simulink model "EPT"  (R2019b)
settings: Solver=FixedStepDiscrete  StartTime=0.0  StopTime=5  FixedStep=0.005  RelTol=1e-3  EnableMultiTasking=on
PreLoadFcn:
  | try, model_open; catch, disp('Error occurred while executing model pre-load callback: model_open.m'); disp('Please assure that the MATLAB working directory is set to the model directory before opening.'); end
InitFcn:
  | try, model_open; catch, end
undefined symbols (not defined in the file or in its folder): Bridge, GCM, H, ln, raptor_get_param_eval, raptor_get_safe_string, raptor_xcp_function
libraries: Raptor_lib x2810, simulink x374, hdlsllib x19
(part 11 of 45)

== system EPT/LED_Status/DualLED_Funny/LED_Status/10Hz ==
  Trigger : TriggerPort  VariantControl=Variant  PortDimensions=1
  NOT : Logic  Operator=NOT  IconShape=distinctive  AllPortsSameDT=off  OutDataTypeStr=boolean
  raptor_data_def : Raptor_lib/Data Storage/raptor_data_def  dataName='Flag_LED_10Hz'  initValue=0  dataType=boolean  storage=Volatile (RAM)  calVisible=on  calType=Measurement  calDispType=Number  calEnum={'False', 'True'}  calGain=1.0  calOffset=0  calMin=-inf  calMax=inf  calFormat='-1'  calUnit=''  calHelp=''  calAccess=1  calFunction=raptor_xcp_function(gcb)  calDispHeaders=off  calColHeaders={'Col1' 'Col2' 'Col3'}  calRowHeaders={'Row1' 'Row2' 'Row3'}
      settings: SourceProductName=Raptor
  raptor_data_read : Raptor_lib/Data Storage/raptor_data_read  dataName='Flag_LED_10Hz'  dataShape=Scalar  idxSource=Input  idxRow=1  idxCol=1
      settings: SourceProductName=Raptor
  raptor_data_write1 : Raptor_lib/Data Storage/raptor_data_write  dataName='Flag_LED_10Hz'  dataShape=Scalar  idxSource=Input Port  idxRow=1  idxCol=1
      settings: SourceProductName=Raptor
  wires:
  NOT/1 -> raptor_data_write1/1
  raptor_data_read/1 -> NOT/1

== system EPT/LED_Status/DualLED_Funny/LED_Status/1Hz ==
  Trigger : TriggerPort  VariantControl=Variant  PortDimensions=1
  NOT : Logic  Operator=NOT  IconShape=distinctive  AllPortsSameDT=off  OutDataTypeStr=boolean
  raptor_data_def : Raptor_lib/Data Storage/raptor_data_def  dataName='Flag_LED_1Hz'  initValue=0  dataType=boolean  storage=Volatile (RAM)  calVisible=on  calType=Measurement  calDispType=Number  calEnum={'False', 'True'}  calGain=1.0  calOffset=0  calMin=-inf  calMax=inf  calFormat='-1'  calUnit=''  calHelp=''  calAccess=1  calFunction=raptor_xcp_function(gcb)  calDispHeaders=off  calColHeaders={'Col1' 'Col2' 'Col3'}  calRowHeaders={'Row1' 'Row2' 'Row3'}
      settings: SourceProductName=Raptor
  raptor_data_read : Raptor_lib/Data Storage/raptor_data_read  dataName='Flag_LED_1Hz'  dataShape=Scalar  idxSource=Input  idxRow=1  idxCol=1
      settings: SourceProductName=Raptor
  raptor_data_write1 : Raptor_lib/Data Storage/raptor_data_write  dataName='Flag_LED_1Hz'  dataShape=Scalar  idxSource=Input Port  idxRow=1  idxCol=1
      settings: SourceProductName=Raptor
  wires:
  raptor_data_read/1 -> NOT/1
  NOT/1 -> raptor_data_write1/1

== system EPT/LED_Status/DualLED_Funny/LED_Status/2Hz ==
  Trigger : TriggerPort  VariantControl=Variant  PortDimensions=1
  NOT : Logic  Operator=NOT  IconShape=distinctive  AllPortsSameDT=off  OutDataTypeStr=boolean
  raptor_data_def : Raptor_lib/Data Storage/raptor_data_def  dataName='Flag_LED_2Hz'  initValue=0  dataType=boolean  storage=Volatile (RAM)  calVisible=on  calType=Measurement  calDispType=Number  calEnum={'False', 'True'}  calGain=1.0  calOffset=0  calMin=-inf  calMax=inf  calFormat='-1'  calUnit=''  calHelp=''  calAccess=1  calFunction=raptor_xcp_function(gcb)  calDispHeaders=off  calColHeaders={'Col1' 'Col2' 'Col3'}  calRowHeaders={'Row1' 'Row2' 'Row3'}
      settings: SourceProductName=Raptor
  raptor_data_read : Raptor_lib/Data Storage/raptor_data_read  dataName='Flag_LED_2Hz'  dataShape=Scalar  idxSource=Input  idxRow=1  idxCol=1
      settings: SourceProductName=Raptor
  raptor_data_write1 : Raptor_lib/Data Storage/raptor_data_write  dataName='Flag_LED_2Hz'  dataShape=Scalar  idxSource=Input Port  idxRow=1  idxCol=1
      settings: SourceProductName=Raptor
  wires:
  NOT/1 -> raptor_data_write1/1
  raptor_data_read/1 -> NOT/1

== system EPT/LED_Status/DualLED_Funny/LED_Status/4Hz ==
  Trigger : TriggerPort  VariantControl=Variant  PortDimensions=1
  NOT : Logic  Operator=NOT  IconShape=distinctive  AllPortsSameDT=off  OutDataTypeStr=boolean
  raptor_data_def : Raptor_lib/Data Storage/raptor_data_def  dataName='Flag_LED_4Hz'  initValue=0  dataType=boolean  storage=Volatile (RAM)  calVisible=on  calType=Measurement  calDispType=Number  calEnum={'False', 'True'}  calGain=1.0  calOffset=0  calMin=-inf  calMax=inf  calFormat='-1'  calUnit=''  calHelp=''  calAccess=1  calFunction=raptor_xcp_function(gcb)  calDispHeaders=off  calColHeaders={'Col1' 'Col2' 'Col3'}  calRowHeaders={'Row1' 'Row2' 'Row3'}
      settings: SourceProductName=Raptor
  raptor_data_read : Raptor_lib/Data Storage/raptor_data_read  dataName='Flag_LED_4Hz'  dataShape=Scalar  idxSource=Input  idxRow=1  idxCol=1
      settings: SourceProductName=Raptor
  raptor_data_write1 : Raptor_lib/Data Storage/raptor_data_write  dataName='Flag_LED_4Hz'  dataShape=Scalar  idxSource=Input Port  idxRow=1  idxCol=1
      settings: SourceProductName=Raptor
  wires:
  raptor_data_read/1 -> NOT/1
  NOT/1 -> raptor_data_write1/1

== system EPT/LED_Status/DualLED_Funny/LED_Status/Alarrn_LED ==
  Action Port : ActionPort  ActionPortLabel=case [ 7 ]:
  Constant1 : Constant  Value=6000
  Constant2 : Constant  Value=0
  Data Type Conversion : DataTypeConversion
  Switch : Switch  Threshold=1
  raptor_data_read : Raptor_lib/Data Storage/raptor_data_read  dataName='Flag_LED_10Hz'  dataShape=Scalar  idxSource=Input  idxRow=1  idxCol=1
      settings: SourceProductName=Raptor
  raptor_data_write : Raptor_lib/Data Storage/raptor_data_write  dataName='LED_Duty'  dataShape=Scalar  idxSource=Input Port  idxRow=1  idxCol=1
      settings: SourceProductName=Raptor
  wires:
  Data Type Conversion/1 -> raptor_data_write/1
  Switch/1 -> Data Type Conversion/1
  Constant2/1 -> Switch/3
  Constant1/1 -> Switch/1
  raptor_data_read/1 -> Switch/2

== system EPT/LED_Status/DualLED_Funny/LED_Status/Charging ==
  Action Port : ActionPort  ActionPortLabel=case [ 1 ]:
  Constant1 : Constant  Value=-6000
  Data Type Conversion : DataTypeConversion
  Product : Product
  raptor_data_read : Raptor_lib/Data Storage/raptor_data_read  dataName='Flag_LED_0_5Hz'  dataShape=Scalar  idxSource=Input  idxRow=1  idxCol=1
      settings: SourceProductName=Raptor
  raptor_data_write : Raptor_lib/Data Storage/raptor_data_write  dataName='LED_Duty'  dataShape=Scalar  idxSource=Input Port  idxRow=1  idxCol=1
      settings: SourceProductName=Raptor
  wires:
  raptor_data_read/1 -> Product/2
  Product/1 -> Data Type Conversion/1
  Constant1/1 -> Product/1
  Data Type Conversion/1 -> raptor_data_write/1

== system EPT/LED_Status/DualLED_Funny/LED_Status/CountTrigger1 ==
  Counter : Inport
  Constant1 : Constant  Value=0
  Constant3 : Constant
  CycleTrigger : Subsystem
  Switch : Switch  Threshold=1
  Unit Delay : UnitDelay  SampleTime=-1  HasFrameUpgradeWarning=on
  Tirgger : Outport  VectorParamsAs1DForOutWhenUnconnected=off
  wires:
  Switch/1 -> CycleTrigger/1(In1)
  Constant3/1 -> Switch/3
  Constant1/1 -> Switch/1
  Counter/1 -> CycleTrigger/2(In2)
  CycleTrigger/1(Trigger) -> Tirgger/1, Unit Delay/1
  Unit Delay/1 -> Switch/2

== system EPT/LED_Status/DualLED_Funny/LED_Status/CountTrigger2 ==
  Counter : Inport
  Constant1 : Constant  Value=0
  Constant3 : Constant
  CycleTrigger : Subsystem
  Switch : Switch  Threshold=1
  Unit Delay : UnitDelay  SampleTime=-1  HasFrameUpgradeWarning=on
  Tirgger : Outport  VectorParamsAs1DForOutWhenUnconnected=off
  wires:
  Unit Delay/1 -> Switch/2
  CycleTrigger/1(Trigger) -> Unit Delay/1, Tirgger/1
  Counter/1 -> CycleTrigger/2(In2)
  Constant1/1 -> Switch/1
  Constant3/1 -> Switch/3
  Switch/1 -> CycleTrigger/1(In1)

== system EPT/LED_Status/DualLED_Funny/LED_Status/CountTrigger3 ==
  Counter : Inport
  Constant1 : Constant  Value=0
  Constant3 : Constant
  CycleTrigger : Subsystem
  Switch : Switch  Threshold=1
  Unit Delay : UnitDelay  SampleTime=-1  HasFrameUpgradeWarning=on
  Tirgger : Outport  VectorParamsAs1DForOutWhenUnconnected=off
  wires:
  Unit Delay/1 -> Switch/2
  CycleTrigger/1(Trigger) -> Unit Delay/1, Tirgger/1
  Counter/1 -> CycleTrigger/2(In2)
  Constant1/1 -> Switch/1
  Constant3/1 -> Switch/3
  Switch/1 -> CycleTrigger/1(In1)

== system EPT/LED_Status/DualLED_Funny/LED_Status/CountTrigger4 ==
  Counter : Inport
  Constant1 : Constant  Value=0
  Constant3 : Constant
  CycleTrigger : Subsystem
  Switch : Switch  Threshold=1
  Unit Delay : UnitDelay  SampleTime=-1  HasFrameUpgradeWarning=on
  Tirgger : Outport  VectorParamsAs1DForOutWhenUnconnected=off
  wires:
  Unit Delay/1 -> Switch/2
  CycleTrigger/1(Trigger) -> Unit Delay/1, Tirgger/1
  Counter/1 -> CycleTrigger/2(In2)
  Constant1/1 -> Switch/1
  Constant3/1 -> Switch/3
  Switch/1 -> CycleTrigger/1(In1)

== system EPT/LED_Status/DualLED_Funny/LED_Status/CountTrigger5 ==
  Counter : Inport
  Constant1 : Constant  Value=0
  Constant3 : Constant
  CycleTrigger : Subsystem
  Switch : Switch  Threshold=1
  Unit Delay : UnitDelay  SampleTime=-1  HasFrameUpgradeWarning=on
  Tirgger : Outport  VectorParamsAs1DForOutWhenUnconnected=off
  wires:
  Switch/1 -> CycleTrigger/1(In1)
  Constant3/1 -> Switch/3
  Constant1/1 -> Switch/1
  Counter/1 -> CycleTrigger/2(In2)
  CycleTrigger/1(Trigger) -> Tirgger/1, Unit Delay/1
  Unit Delay/1 -> Switch/2

== system EPT/LED_Status/DualLED_Funny/LED_Status/CountTrigger6 ==
  Counter : Inport
  Constant1 : Constant  Value=0
  Constant3 : Constant
  CycleTrigger : Subsystem
  Switch : Switch  Threshold=1
  Unit Delay : UnitDelay  SampleTime=-1  HasFrameUpgradeWarning=on
  Tirgger : Outport  VectorParamsAs1DForOutWhenUnconnected=off
  wires:
  Switch/1 -> CycleTrigger/1(In1)
  Constant3/1 -> Switch/3
  Constant1/1 -> Switch/1
  Counter/1 -> CycleTrigger/2(In2)
  CycleTrigger/1(Trigger) -> Tirgger/1, Unit Delay/1
  Unit Delay/1 -> Switch/2

== system EPT/LED_Status/DualLED_Funny/LED_Status/D  ==
  Action Port : ActionPort  ActionPortLabel=case [ 6 ]:
  Abs : Abs
  Add1 : Sum
  Compare To Constant : simulink/Logic and Bit Operations/Compare To Constant  relop=>=  const=6000  OutDataTypeStr=boolean
  Compare To Constant1 : simulink/Logic and Bit Operations/Compare To Constant  relop=<=  const=-6000  OutDataTypeStr=boolean
  Data Type Conversion : DataTypeConversion
  Data Type Conversion1 : DataTypeConversion
  Gain2 : Gain  Gain=-1
  If1 : If  IfExpression=u1 >= 1  ShowElse=off
  Logical Operator : Logic  Operator=OR  AllPortsSameDT=off  OutDataTypeStr=boolean
  Scope1 : Scope
  Switch : Switch  Threshold=1
  Transition state : Subsystem  TreatAsAtomicUnit=on
  Unit Delay : UnitDelay  SampleTime=-1  HasFrameUpgradeWarning=on
  raptor_adjustment : Raptor_lib/Data Storage/raptor_adjustment  paramName='Cal_D_Duty_Scale'  nameSource=Parameter  initValue=30  dataType=double  storage=Calibration  calDispType=Number  calEnum={'False', 'True'}  calGain=1.0  calOffset=0.0  calMax=inf  calMin=-inf  calFormat='-1'  calUnit=''  calHelp=''  calAccess=1  calFunction=raptor_xcp_function(gcb)  calDispHeaders=off  calColHeaders={'Col1' 'Col2' 'Col3'}  calRowHeaders={'Row1' 'Row2' 'Row3'}
      settings: SourceProductName=Raptor
  raptor_data_read : Raptor_lib/Data Storage/raptor_data_read  dataName='LED_Gradient'  dataShape=Scalar  idxSource=Input  idxRow=1  idxCol=1
      settings: SourceProductName=Raptor
  raptor_data_write : Raptor_lib/Data Storage/raptor_data_write  dataName='LED_Duty'  dataShape=Scalar  idxSource=Input Port  idxRow=1  idxCol=1
      settings: SourceProductName=Raptor
  wires:
  Abs/1 -> Data Type Conversion/1
  If1/1 -> Transition state/Action
  Compare To Constant/1 -> Logical Operator/1
  Switch/1 -> Add1/2
  Compare To Constant1/1 -> Logical Operator/2
  Gain2/1 -> Switch/1
  Add1/1 -> Compare To Constant/1, Compare To Constant1/1, Scope1/1, Unit Delay/1, Abs/1
  raptor_adjustment/1 -> Gain2/1, Switch/3
  Data Type Conversion/1 -> raptor_data_write/1
  raptor_data_read/1 -> Switch/2
  Logical Operator/1 -> Data Type Conversion1/1
  Unit Delay/1 -> Add1/1
  Data Type Conversion1/1 -> If1/1

== system EPT/LED_Status/DualLED_Funny/LED_Status/EVSE Conected ==
  Action Port : ActionPort  ActionPortLabel=case [ 2 ]:
  Abs : Abs
  Add1 : Sum
  Compare To Constant : simulink/Logic and Bit Operations/Compare To Constant  relop=>=  const=6000  OutDataTypeStr=boolean
  Compare To Constant1 : simulink/Logic and Bit Operations/Compare To Constant  relop=<=  const=-6000  OutDataTypeStr=boolean
  Constant5 : Constant  Value=30
  Data Type Conversion : DataTypeConversion
  Data Type Conversion1 : DataTypeConversion
  Gain1 : Gain  Gain=-1
  Gain2 : Gain  Gain=-1
  If1 : If  IfExpression=u1 >= 1  ShowElse=off
  Logical Operator : Logic  Operator=OR  AllPortsSameDT=off  OutDataTypeStr=boolean
  Scope1 : Scope
  Switch : Switch  Threshold=1
  Transition state : Subsystem  TreatAsAtomicUnit=on
  Unit Delay : UnitDelay  SampleTime=-1  HasFrameUpgradeWarning=on
  raptor_data_read : Raptor_lib/Data Storage/raptor_data_read  dataName='LED_Gradient'  dataShape=Scalar  idxSource=Input  idxRow=1  idxCol=1
      settings: SourceProductName=Raptor
  raptor_data_write : Raptor_lib/Data Storage/raptor_data_write  dataName='LED_Duty'  dataShape=Scalar  idxSource=Input Port  idxRow=1  idxCol=1
      settings: SourceProductName=Raptor
  wires:
  Gain1/1 -> Data Type Conversion/1
  Data Type Conversion/1 -> raptor_data_write/1
  Abs/1 -> Gain1/1
  Compare To Constant1/1 -> Logical Operator/2
  Constant5/1 -> Gain2/1, Switch/3
  Gain2/1 -> Switch/1
  Add1/1 -> Compare To Constant/1, Compare To Constant1/1, Scope1/1, Unit Delay/1, Abs/1
  Unit Delay/1 -> Add1/1
  Logical Operator/1 -> Data Type Conversion1/1
  raptor_data_read/1 -> Switch/2
  Compare To Constant/1 -> Logical Operator/1
  If1/1 -> Transition state/Action
  Switch/1 -> Add1/2
  Data Type Conversion1/1 -> If1/1

== system EPT/LED_Status/DualLED_Funny/LED_Status/N ==
  Action Port : ActionPort  ActionPortLabel=case [ 5 ]:
  Constant1 : Constant  Value=6000
  Data Type Conversion : DataTypeConversion
  Product : Product  Inputs=3
  raptor_data_read : Raptor_lib/Data Storage/raptor_data_read  dataName='Flag_LED_0_5Hz'  dataShape=Scalar  idxSource=Input  idxRow=1  idxCol=1
      settings: SourceProductName=Raptor
  raptor_data_read1 : Raptor_lib/Data Storage/raptor_data_read  dataName='Flag_LED_2Hz'  dataShape=Scalar  idxSource=Input  idxRow=1  idxCol=1
      settings: SourceProductName=Raptor
  raptor_data_write : Raptor_lib/Data Storage/raptor_data_write  dataName='LED_Duty'  dataShape=Scalar  idxSource=Input Port  idxRow=1  idxCol=1
      settings: SourceProductName=Raptor
  wires:
  raptor_data_read/1 -> Product/2
  Product/1 -> Data Type Conversion/1
  Constant1/1 -> Product/1
  Data Type Conversion/1 -> raptor_data_write/1
  raptor_data_read1/1 -> Product/3

== system EPT/LED_Status/DualLED_Funny/LED_Status/No Mode ==
  Action Port : ActionPort  ActionPortLabel=case [ 0 ]:
  Data Type Conversion : DataTypeConversion
  Switch : Switch  Criteria=u2 > Threshold
  raptor_adjustment : Raptor_lib/Data Storage/raptor_adjustment  paramName='Cal_No_Mode_G'  nameSource=Parameter  initValue=-1000  dataType=double  storage=Calibration  calDispType=Number  calEnum={'False', 'True'}  calGain=1.0  calOffset=0.0  calMax=inf  calMin=-inf  calFormat='-1'  calUnit=''  calHelp=''  calAccess=1  calFunction=raptor_xcp_function(gcb)  calDispHeaders=off  calColHeaders={'Col1' 'Col2' 'Col3'}  calRowHeaders={'Row1' 'Row2' 'Row3'}
      settings: SourceProductName=Raptor
  raptor_adjustment1 : Raptor_lib/Data Storage/raptor_adjustment  paramName='Cal_No_Mode_R'  nameSource=Parameter  initValue=3000  dataType=double  storage=Calibration  calDispType=Number  calEnum={'False', 'True'}  calGain=1.0  calOffset=0.0  calMax=inf  calMin=-inf  calFormat='-1'  calUnit=''  calHelp=''  calAccess=1  calFunction=raptor_xcp_function(gcb)  calDispHeaders=off  calColHeaders={'Col1' 'Col2' 'Col3'}  calRowHeaders={'Row1' 'Row2' 'Row3'}
      settings: SourceProductName=Raptor
  raptor_data_read : Raptor_lib/Data Storage/raptor_data_read  dataName='Flag_LED_100Hz'  dataShape=Scalar  idxSource=Input  idxRow=1  idxCol=1
      settings: SourceProductName=Raptor
  raptor_data_write : Raptor_lib/Data Storage/raptor_data_write  dataName='LED_Duty'  dataShape=Scalar  idxSource=Input Port  idxRow=1  idxCol=1
      settings: SourceProductName=Raptor
  wires:
  Data Type Conversion/1 -> raptor_data_write/1
  Switch/1 -> Data Type Conversion/1
  raptor_adjustment/1 -> Switch/1
  raptor_adjustment1/1 -> Switch/3
  raptor_data_read/1 -> Switch/2

== system EPT/LED_Status/DualLED_Funny/LED_Status/P ==
  Action Port : ActionPort  ActionPortLabel=case [ 3 ]:
  Constant1 : Constant  Value=6000
  Data Type Conversion : DataTypeConversion
  Product : Product
  raptor_data_read : Raptor_lib/Data Storage/raptor_data_read  dataName='Flag_LED_0_5Hz'  dataShape=Scalar  idxSource=Input  idxRow=1  idxCol=1
      settings: SourceProductName=Raptor
  raptor_data_write : Raptor_lib/Data Storage/raptor_data_write  dataName='LED_Duty'  dataShape=Scalar  idxSource=Input Port  idxRow=1  idxCol=1
      settings: SourceProductName=Raptor
  wires:
  Data Type Conversion/1 -> raptor_data_write/1
  Constant1/1 -> Product/1
  Product/1 -> Data Type Conversion/1
  raptor_data_read/1 -> Product/2

== system EPT/LED_Status/DualLED_Funny/LED_Status/R ==
  Action Port : ActionPort  ActionPortLabel=case [ 4 ]:
  Abs : Abs
  Add1 : Sum
  Add2 : Sum
  Compare To Constant : simulink/Logic and Bit Operations/Compare To Constant  relop=>=  const=6000  OutDataTypeStr=boolean
  Compare To Constant1 : simulink/Logic and Bit Operations/Compare To Constant  relop=<=  const=3000  OutDataTypeStr=boolean
  Data Type Conversion : DataTypeConversion
  Data Type Conversion1 : DataTypeConversion
  Gain2 : Gain  Gain=-1
  If1 : If  IfExpression=u1 >= 1  ShowElse=off
  Logical Operator : Logic  Operator=OR  AllPortsSameDT=off  OutDataTypeStr=boolean
  Scope1 : Scope
  Switch : Switch  Threshold=1
  Transition state : Subsystem  TreatAsAtomicUnit=on
  Unit Delay : UnitDelay  SampleTime=-1  HasFrameUpgradeWarning=on
  raptor_adjustment : Raptor_lib/Data Storage/raptor_adjustment  paramName='Cal_R_Duty_Scale'  nameSource=Parameter  initValue=100  dataType=double  storage=Calibration  calDispType=Number  calEnum={'False', 'True'}  calGain=1.0  calOffset=0.0  calMax=inf  calMin=-inf  calFormat='-1'  calUnit=''  calHelp=''  calAccess=1  calFunction=raptor_xcp_function(gcb)  calDispHeaders=off  calColHeaders={'Col1' 'Col2' 'Col3'}  calRowHeaders={'Row1' 'Row2' 'Row3'}
      settings: SourceProductName=Raptor
  raptor_adjustment1 : Raptor_lib/Data Storage/raptor_adjustment  paramName='Cal_R_Base_Duty'  nameSource=Parameter  initValue=1000  dataType=double  storage=Calibration  calDispType=Number  calEnum={'False', 'True'}  calGain=1.0  calOffset=0.0  calMax=inf  calMin=-inf  calFormat='-1'  calUnit=''  calHelp=''  calAccess=1  calFunction=raptor_xcp_function(gcb)  calDispHeaders=off  calColHeaders={'Col1' 'Col2' 'Col3'}  calRowHeaders={'Row1' 'Row2' 'Row3'}
      settings: SourceProductName=Raptor
  raptor_data_read : Raptor_lib/Data Storage/raptor_data_read  dataName='LED_Gradient'  dataShape=Scalar  idxSource=Input  idxRow=1  idxCol=1
      settings: SourceProductName=Raptor
  raptor_data_write : Raptor_lib/Data Storage/raptor_data_write  dataName='LED_Duty'  dataShape=Scalar  idxSource=Input Port  idxRow=1  idxCol=1
      settings: SourceProductName=Raptor
  wires:
  Data Type Conversion1/1 -> If1/1
  Unit Delay/1 -> Add1/1
  Logical Operator/1 -> Data Type Conversion1/1
  raptor_data_read/1 -> Switch/2
  raptor_adjustment/1 -> Switch/3, Gain2/1
  Add1/1 -> Add2/1, Unit Delay/1, Scope1/1
  Gain2/1 -> Switch/1
  Compare To Constant1/1 -> Logical Operator/2
  Switch/1 -> Add1/2
  Compare To Constant/1 -> Logical Operator/1
  If1/1 -> Transition state/Action
  Abs/1 -> Data Type Conversion/1
  Data Type Conversion/1 -> raptor_data_write/1
  Add2/1 -> Compare To Constant1/1, Compare To Constant/1, Abs/1
  raptor_adjustment1/1 -> Add2/2

== system EPT/Power Up_Down/Background/Store EEPROM Value/Subsystem ==
  Enable : EnablePort
  Add : Sum
  Constant : Constant
  raptor_data_read1 : Raptor_lib/Data Storage/raptor_data_read  dataName='EEPROM_CountTest'  dataShape=Scalar  idxSource=Input  idxRow=1  idxCol=1
      settings: SourceProductName=Raptor
  raptor_data_read2 : Raptor_lib/Data Storage/raptor_data_read  dataName='EPT_BPOBU_RCAP'  dataShape=Scalar  idxSource=Input  idxRow=1  idxCol=1
      settings: SourceProductName=Raptor
  raptor_data_write1 : Raptor_lib/Data Storage/raptor_data_write  dataName='EEPROM_RCAP'  dataShape=Scalar  idxSource=Input Port  idxRow=1  idxCol=1
      settings: SourceProductName=Raptor
  raptor_data_write2 : Raptor_lib/Data Storage/raptor_data_write  dataName='EEPROM_Count'  dataShape=Scalar  idxSource=Input Port  idxRow=1  idxCol=1
      settings: SourceProductName=Raptor
  wires:
  Constant/1 -> Add/2
  Add/1 -> raptor_data_write2/1
  raptor_data_read1/1 -> Add/1
  raptor_data_read2/1 -> raptor_data_write1/1

== system EPT/Power Up_Down/Background/Store EEPROM Value/Subsystem1 ==
  Enable : EnablePort
  raptor_data_read2 : Raptor_lib/Data Storage/raptor_data_read  dataName='DOD_t'  dataShape=Scalar  idxSource=Input  idxRow=1  idxCol=1
      settings: SourceProductName=Raptor
  raptor_data_write1 : Raptor_lib/Data Storage/raptor_data_write  dataName='EEPROM_DOD_t0'  dataShape=Scalar  idxSource=Input Port  idxRow=1  idxCol=1
      settings: SourceProductName=Raptor
  wires:
  raptor_data_read2/1 -> raptor_data_write1/1

== system EPT/Power Up_Down/Background/Store EEPROM Value/Subsystem2 ==
  Enable : EnablePort
  raptor_data_read2 : Raptor_lib/Data Storage/raptor_data_read  dataName='New_SOH'  dataShape=Scalar  idxSource=Input  idxRow=1  idxCol=1
      settings: SourceProductName=Raptor
  raptor_data_write1 : Raptor_lib/Data Storage/raptor_data_write  dataName='EEPROM_SOH'  dataShape=Scalar  idxSource=Input Port  idxRow=1  idxCol=1
      settings: SourceProductName=Raptor
  wires:
  raptor_data_read2/1 -> raptor_data_write1/1

== system EPT/Power Up_Down/Background/Store EEPROM Value/Subsystem3 ==
  Enable : EnablePort
  raptor_data_read2 : Raptor_lib/Data Storage/raptor_data_read  dataName='EPT_BPOBU_FCCAP'  dataShape=Scalar  idxSource=Input  idxRow=1  idxCol=1
      settings: SourceProductName=Raptor
  raptor_data_write1 : Raptor_lib/Data Storage/raptor_data_write  dataName='EEPROM_FCCAP'  dataShape=Scalar  idxSource=Input Port  idxRow=1  idxCol=1
      settings: SourceProductName=Raptor
  wires:
  raptor_data_read2/1 -> raptor_data_write1/1

== system EPT/Test/Coulomb Counting Method Test/5ms/CountTrigger3 ==
  Counter : Inport
  Constant1 : Constant  Value=0
  Constant3 : Constant
  CycleTrigger : Subsystem
  Switch : Switch  Threshold=1
  Unit Delay1 : UnitDelay  SampleTime=-1  HasFrameUpgradeWarning=on
  Unit Delay2 : UnitDelay  SampleTime=-1  HasFrameUpgradeWarning=on
  Tirgger : Outport  VectorParamsAs1DForOutWhenUnconnected=off
  wires:
  Switch/1 -> Unit Delay1/1
  Constant3/1 -> Switch/3
  Constant1/1 -> Switch/1
  Counter/1 -> CycleTrigger/2(In2)
  CycleTrigger/1(Trigger) -> Switch/2, Unit Delay2/1
  Unit Delay1/1 -> CycleTrigger/1(In1)
  Unit Delay2/1 -> Tirgger/1

== system EPT/Test/Coulomb Counting Method Test/5ms/CountTrigger4 ==
  Counter : Inport
  Constant1 : Constant  Value=0
  Constant3 : Constant
  CycleTrigger : Subsystem
  Switch : Switch  Threshold=1
  Unit Delay1 : UnitDelay  SampleTime=-1  HasFrameUpgradeWarning=on
  Unit Delay2 : UnitDelay  SampleTime=-1  HasFrameUpgradeWarning=on
  Tirgger : Outport  VectorParamsAs1DForOutWhenUnconnected=off
  wires:
  Unit Delay2/1 -> Tirgger/1
  Unit Delay1/1 -> CycleTrigger/1(In1)
  CycleTrigger/1(Trigger) -> Unit Delay2/1, Switch/2
  Counter/1 -> CycleTrigger/2(In2)
  Constant1/1 -> Switch/1
  Constant3/1 -> Switch/3
  Switch/1 -> Unit Delay1/1

== system EPT/Test/Coulomb Counting Method Test/CountTrigger/CycleTrigger ==
  In1 : Inport
  In2 : Inport  Port=2
  Add : Sum
  Add2 : Sum  Inputs=+-
  Constant2 : Constant  Value=0
  Constant3 : Constant
  Data Type Conversion1 : DataTypeConversion
  Data Type Conversion2 : DataTypeConversion
  Relational Operator1 : RelationalOperator  OutDataTypeStr=boolean  RndMeth=Simplest
  Scope1 : Scope
  Scope2 : Scope
  Switch : Switch  Threshold=1
  Unit Delay : UnitDelay  SampleTime=-1  HasFrameUpgradeWarning=on
  Trigger : Outport  VectorParamsAs1DForOutWhenUnconnected=off
  wires:
  Add/1 -> Switch/1
  In1/1 -> Data Type Conversion2/1
  Unit Delay/1 -> Add/1
  Switch/1 -> Relational Operator1/1, Scope1/1, Unit Delay/1
  Relational Operator1/1 -> Scope2/1, Trigger/1
  Data Type Conversion1/1 -> Relational Operator1/2
  Constant2/1 -> Switch/3
  Data Type Conversion2/1 -> Add/2, Switch/2
  Add2/1 -> Data Type Conversion1/1
  In2/1 -> Add2/1
  Constant3/1 -> Add2/2

== system EPT/Test/DualLEDTest/GreenBreath/Transition state ==
  Action Port : ActionPort
  NOT : Logic  Operator=NOT  IconShape=distinctive  AllPortsSameDT=off  OutDataTypeStr=boolean
  raptor_data_read : Raptor_lib/Data Storage/raptor_data_read  dataName='LED_Gradient'  dataShape=Scalar  idxSource=Input  idxRow=1  idxCol=1
      settings: SourceProductName=Raptor
  raptor_data_write : Raptor_lib/Data Storage/raptor_data_write  dataName='LED_Gradient'  dataShape=Scalar  idxSource=Input Port  idxRow=1  idxCol=1
      settings: SourceProductName=Raptor
  wires:
  NOT/1 -> raptor_data_write/1
  raptor_data_read/1 -> NOT/1

== system EPT/Test/DualLEDTest/RedBreath/Transition state ==
  Action Port : ActionPort
  NOT : Logic  Operator=NOT  IconShape=distinctive  AllPortsSameDT=off  OutDataTypeStr=boolean
  raptor_data_read : Raptor_lib/Data Storage/raptor_data_read  dataName='LED_Gradient'  dataShape=Scalar  idxSource=Input  idxRow=1  idxCol=1
      settings: SourceProductName=Raptor
  raptor_data_write : Raptor_lib/Data Storage/raptor_data_write  dataName='LED_Gradient'  dataShape=Scalar  idxSource=Input Port  idxRow=1  idxCol=1
      settings: SourceProductName=Raptor
  wires:
  NOT/1 -> raptor_data_write/1
  raptor_data_read/1 -> NOT/1

== system EPT/Test/LED For CMU/deBounce 2/CycleTrigger1 ==
  In1 : Inport
  In2 : Inport  Port=2
  Add : Sum
  Add1 : Sum
  Add2 : Sum  Inputs=+-
  Constant1 : Constant
  Constant2 : Constant  Value=0
  Constant3 : Constant
  Data Type Conversion1 : DataTypeConversion
  Data Type Conversion2 : DataTypeConversion
  Display : Display
  Relational Operator1 : RelationalOperator  OutDataTypeStr=boolean  RndMeth=Simplest
  Saturation : Saturate  UpperLimit=inf  LowerLimit=2
  Scope : Scope
  Scope1 : Scope
  Scope2 : Scope
  Switch : Switch  Threshold=1
  Unit Delay : UnitDelay  SampleTime=-1  HasFrameUpgradeWarning=on
  Unit Delay1 : UnitDelay  SampleTime=-1  HasFrameUpgradeWarning=on
  Trigger : Outport  VectorParamsAs1DForOutWhenUnconnected=off
  wires:
  Constant3/1 -> Add2/2
  In2/1 -> Saturation/1
  Add2/1 -> Data Type Conversion1/1
  Data Type Conversion2/1 -> Switch/2, Add/2
  Constant2/1 -> Switch/3
  Data Type Conversion1/1 -> Relational Operator1/2
  Relational Operator1/1 -> Trigger/1, Scope2/1
  Constant1/1 -> Add1/2
  Unit Delay1/1 -> Add1/1
  Add1/1 -> Display/1, Unit Delay1/1, Scope/1
  Switch/1 -> Unit Delay/1, Scope1/1, Relational Operator1/1
  Unit Delay/1 -> Add/1
  In1/1 -> Data Type Conversion2/1
  Add/1 -> Switch/1
  Saturation/1 -> Add2/1

== system EPT/Test/LifeCycleTest/LifeCycleDetect/Latch1 ==
  Latch : Inport
  Reset : Inport  Port=2
  Switch1 : Switch  Criteria=u2 > Threshold
  Switch3 : Switch  Criteria=u2 > Threshold
  Unit Delay1 : UnitDelay  SampleTime=-1  HasFrameUpgradeWarning=on
  Output : Outport  VectorParamsAs1DForOutWhenUnconnected=off
  wires:
  Unit Delay1/1 -> Switch1/3
  Switch3/1 -> Output/1, Unit Delay1/1
  Reset/1 -> Switch3/2
  Latch/1 -> Switch1/1, Switch1/2
  Switch1/1 -> Switch3/3

== system EPT/Test/RPB1600_Read/CountTrigger/CycleTrigger ==
  In1 : Inport
  In2 : Inport  Port=2
  Add : Sum
  Add1 : Sum
  Add2 : Sum  Inputs=+-
  Constant1 : Constant
  Constant2 : Constant  Value=0
  Constant3 : Constant
  Data Type Conversion1 : DataTypeConversion
  Data Type Conversion2 : DataTypeConversion
  Display : Display
  Relational Operator1 : RelationalOperator  OutDataTypeStr=boolean  RndMeth=Simplest
  Scope : Scope
  Scope1 : Scope
  Scope2 : Scope
  Switch : Switch  Threshold=1
  Unit Delay : UnitDelay  SampleTime=-1  HasFrameUpgradeWarning=on
  Unit Delay1 : UnitDelay  SampleTime=-1  HasFrameUpgradeWarning=on
  Trigger : Outport  VectorParamsAs1DForOutWhenUnconnected=off
  wires:
  Constant3/1 -> Add2/2
  In2/1 -> Add2/1
  Add2/1 -> Data Type Conversion1/1
  Data Type Conversion2/1 -> Switch/2, Add/2
  Constant2/1 -> Switch/3
  Data Type Conversion1/1 -> Relational Operator1/2
  Relational Operator1/1 -> Trigger/1, Scope2/1
  Constant1/1 -> Add1/2
  Unit Delay1/1 -> Add1/1
  Add1/1 -> Display/1, Unit Delay1/1, Scope/1
  Switch/1 -> Unit Delay/1, Scope1/1, Relational Operator1/1
  Unit Delay/1 -> Add/1
  In1/1 -> Data Type Conversion2/1
  Add/1 -> Switch/1

== system EPT/Test/RPB1600_Read/RPB1600_RX_20ms/Convert_Byte2Data ==
  LowByte : Inport
  HighByte : Inport  Port=2
  Offset : Inport  Port=3
  Factor : Inport  Port=4
  Add2 : Sum
  Add5 : Sum
  Constant10 : Constant  Value=256
  Data Type Conversion10 : DataTypeConversion
  Divide6 : Product  Inputs=**
  Divide9 : Product  Inputs=**
  Data(int16) : Outport  VectorParamsAs1DForOutWhenUnconnected=off
  wires:
  Divide6/1 -> Add2/2
  LowByte/1 -> Add2/1
  Divide9/1 -> Data Type Conversion10/1
  HighByte/1 -> Divide6/1
  Constant10/1 -> Divide6/2
  Add5/1 -> Divide9/1
  Add2/1 -> Add5/1
  Data Type Conversion10/1 -> Data(int16)/1
  Offset/1 -> Add5/2
  Factor/1 -> Divide9/2

== system EPT/Test/RPB1600_Read/RPB1600_RX_20ms/Subsystem ==
  Rx Data : Inport
  Task Input : Inport  Port=2
  "Task Set " : Inport  Port=3
  Delay : Delay  DelayLength=1
  Relational Operator : RelationalOperator  Operator===  OutDataTypeStr=boolean  RndMeth=Simplest
  Switch : Switch  Criteria=u2 > Threshold
  Output : Outport  VectorParamsAs1DForOutWhenUnconnected=off
  wires:
  Relational Operator/1 -> Switch/2
  Switch/1 -> Output/1, Delay/1
  Delay/1 -> Switch/3
  "Task Set "/1 -> Relational Operator/2
  Task Input/1 -> Relational Operator/1
  Rx Data/1 -> Switch/1

== system EPT/Test/RPB1600_Read/RPB1600_RX_20ms/Subsystem1 ==
  Rx Data : Inport
  Task Input : Inport  Port=2
  "Task Set " : Inport  Port=3
  Delay : Delay  DelayLength=1
  Relational Operator : RelationalOperator  Operator===  OutDataTypeStr=boolean  RndMeth=Simplest
  Switch : Switch  Criteria=u2 > Threshold
  Output : Outport  VectorParamsAs1DForOutWhenUnconnected=off
  wires:
  Rx Data/1 -> Switch/1
  Task Input/1 -> Relational Operator/1
  "Task Set "/1 -> Relational Operator/2
  Delay/1 -> Switch/3
  Switch/1 -> Delay/1, Output/1
  Relational Operator/1 -> Switch/2

== system EPT/Test/RPB1600_Read/RPB1600_RX_20ms/Subsystem2 ==
  Rx Data : Inport
  Task Input : Inport  Port=2
  "Task Set " : Inport  Port=3
  Delay : Delay  DelayLength=1
  Relational Operator : RelationalOperator  Operator===  OutDataTypeStr=boolean  RndMeth=Simplest
  Switch : Switch  Criteria=u2 > Threshold
  Output : Outport  VectorParamsAs1DForOutWhenUnconnected=off
  wires:
  Relational Operator/1 -> Switch/2
  Switch/1 -> Output/1, Delay/1
  Delay/1 -> Switch/3
  "Task Set "/1 -> Relational Operator/2
  Task Input/1 -> Relational Operator/1
  Rx Data/1 -> Switch/1

== system EPT/Test/RPB1600_Read/RPB1600_RX_20ms/Subsystem3 ==
  Rx Data : Inport
  Task Input : Inport  Port=2
  "Task Set " : Inport  Port=3
  Delay : Delay  DelayLength=1
  Relational Operator : RelationalOperator  Operator===  OutDataTypeStr=boolean  RndMeth=Simplest
  Switch : Switch  Criteria=u2 > Threshold
  Output : Outport  VectorParamsAs1DForOutWhenUnconnected=off
  wires:
  Rx Data/1 -> Switch/1
  Task Input/1 -> Relational Operator/1
  "Task Set "/1 -> Relational Operator/2
  Delay/1 -> Switch/3
  Switch/1 -> Delay/1, Output/1
  Relational Operator/1 -> Switch/2

== system EPT/Test/RPB1600_Read/RPB1600_RX_20ms/Subsystem4 ==
  Rx Data : Inport
  Task Input : Inport  Port=2
  "Task Set " : Inport  Port=3
  Delay : Delay  DelayLength=1
  Relational Operator : RelationalOperator  Operator===  OutDataTypeStr=boolean  RndMeth=Simplest
  Switch : Switch  Criteria=u2 > Threshold
  Output : Outport  VectorParamsAs1DForOutWhenUnconnected=off
  wires:
  Relational Operator/1 -> Switch/2
  Switch/1 -> Output/1, Delay/1
  Delay/1 -> Switch/3
  "Task Set "/1 -> Relational Operator/2
  Task Input/1 -> Relational Operator/1
  Rx Data/1 -> Switch/1

== system EPT/Test/RPB1600_Read/RPB1600_RX_20ms/Subsystem5 ==
  Rx Data : Inport
  Task Input : Inport  Port=2
  "Task Set " : Inport  Port=3
  Delay : Delay  DelayLength=1
  Relational Operator : RelationalOperator  Operator===  OutDataTypeStr=boolean  RndMeth=Simplest
  Switch : Switch  Criteria=u2 > Threshold
  Output : Outport  VectorParamsAs1DForOutWhenUnconnected=off
  wires:
  Rx Data/1 -> Switch/1
  Task Input/1 -> Relational Operator/1
  "Task Set "/1 -> Relational Operator/2
  Delay/1 -> Switch/3
  Switch/1 -> Delay/1, Output/1
  Relational Operator/1 -> Switch/2

== system EPT/Test/RPB1600_Read/RPB1600_RX_20ms/Subsystem6 ==
  Rx Data : Inport
  Task Input : Inport  Port=2
  "Task Set " : Inport  Port=3
  Delay : Delay  DelayLength=1
  Relational Operator : RelationalOperator  Operator===  OutDataTypeStr=boolean  RndMeth=Simplest
  Switch : Switch  Criteria=u2 > Threshold
  Output : Outport  VectorParamsAs1DForOutWhenUnconnected=off
  wires:
  Relational Operator/1 -> Switch/2
  Switch/1 -> Output/1, Delay/1
  Delay/1 -> Switch/3
  "Task Set "/1 -> Relational Operator/2
  Task Input/1 -> Relational Operator/1
  Rx Data/1 -> Switch/1

== system EPT/Test/RPB1600_Read/RPB1600_RX_20ms/Subsystem7 ==
  Rx Data : Inport
  Task Input : Inport  Port=2
  "Task Set " : Inport  Port=3
  Delay : Delay  DelayLength=1
  Relational Operator : RelationalOperator  Operator===  OutDataTypeStr=boolean  RndMeth=Simplest
  Switch : Switch  Criteria=u2 > Threshold
  Output : Outport  VectorParamsAs1DForOutWhenUnconnected=off
  wires:
  Rx Data/1 -> Switch/1
  Task Input/1 -> Relational Operator/1
  "Task Set "/1 -> Relational Operator/2
  Delay/1 -> Switch/3
  Switch/1 -> Delay/1, Output/1
  Relational Operator/1 -> Switch/2

== system EPT/Test/RPB1600_Read/RPB1600_RX_20ms/Subsystem8 ==
  Rx Data : Inport
  Task Input : Inport  Port=2
  "Task Set " : Inport  Port=3
  Delay : Delay  DelayLength=1
  Relational Operator : RelationalOperator  Operator===  OutDataTypeStr=boolean  RndMeth=Simplest
  Switch : Switch  Criteria=u2 > Threshold
  Output : Outport  VectorParamsAs1DForOutWhenUnconnected=off
  wires:
  Relational Operator/1 -> Switch/2
  Switch/1 -> Output/1, Delay/1
  Delay/1 -> Switch/3
  "Task Set "/1 -> Relational Operator/2
  Task Input/1 -> Relational Operator/1
  Rx Data/1 -> Switch/1

== system EPT/Test/RPB1600_Read/RPB1600_RX_20ms/Subsystem9 ==
  Rx Data : Inport
  Task Input : Inport  Port=2
  "Task Set " : Inport  Port=3
  Delay : Delay  DelayLength=1
  Relational Operator : RelationalOperator  Operator===  OutDataTypeStr=boolean  RndMeth=Simplest
  Switch : Switch  Criteria=u2 > Threshold
  Output : Outport  VectorParamsAs1DForOutWhenUnconnected=off
  wires:
  Rx Data/1 -> Switch/1
  Task Input/1 -> Relational Operator/1
  "Task Set "/1 -> Relational Operator/2
  Delay/1 -> Switch/3
  Switch/1 -> Delay/1, Output/1
  Relational Operator/1 -> Switch/2

== system EPT/Test/RPB1600_Read/RPB1600_RX_20ms/Task Rolling ==
  Constant : Constant  Value=9
  RollingCount : Subsystem
  raptor_data_write : Raptor_lib/Data Storage/raptor_data_write  dataName='RPB1600_Task'  dataShape=Scalar  idxSource=Input Port  idxRow=1  idxCol=1
      settings: SourceProductName=Raptor
  wires:
  Constant/1 -> RollingCount/1(In1)
  RollingCount/1(Out1) -> raptor_data_write/1

== system EPT/Foreground_TimeBase_5ms/CAN/CAN1_exec/BCU vs RMDA-BMS/BCU-OBU Output-CTL  ==
  Trigger : TriggerPort  VariantControl=Variant  PortDimensions=1
  raptor_can_txmsg : Raptor_lib/CAN/raptor_can_txmsg  canDefinition=struct('dbcFile', 'BCU_OBU_HMI.dbc','message', 'BCU_OBU_OutputCTL','comment', '','signals', {{'BP_OBU_Vchg_EXP','BP_OBU_Ichg_EXP','BP_OBU_Iregen_LC','BP_OBU_Idchg_LC','BP_OBU_min_Limit','BP_OBU_Vmax_Limit'}},'enabled', [ 1 1 1 1 1 1;],'canBus', '''CAN1''','messageID', [ 1529;],'idMask', [ 536870911;],'payloadMask', [],'payloadValue', [],'period', [ 0;],'mailbox', '','queueSize', [ 1;],'label', [ 0;],'ver', [ 2;],'showID', [ 0;],'showRaw', [ 0;],'fill', [ 0;],'editID', [ 0;],'signalOrder', [ 2;])  canBus='CAN1'  queueSize=1  payloadMask=[]  payloadValue=[]  period=0  showID=0  label=0  idMask=hex2dec('1FFFFFFF')  fill=0  id=1529  showRaw=0  signalOrder=2  signalInfo={{struct('Name', 'BP_OBU_Vmax_Limit','Startbit', [ 0;],'SignalSize', [ 16;],'ByteOrder', 'BigEndian','ValueType', 'UNSIGNED','Class', 'uint16','Signed', [ 0;],'Factor', [ 0.01;],'Offset', [ 0;],'Min', [ 0;],'Max', [ 0;],'Units', '','Comment', '','StartBit', [ 8;]),struct('Name', 'BP_OBU_min_Limit','Startbit', [ 0;],'SignalSize', [ 16;],'ByteOrder', 'BigEndian','ValueType', 'UNSIGNED','Class', 'uint16','Signed', [ 0;],'Factor', [ 0.01;],'Offset', [ 0;],'Min', [ 0;],'Max', [ 0;],'Units', '','Comment', '','StartBit', [ 24;]),struct('Name', 'BP_OBU_Idchg_LC','Startbit', [ 0;],'SignalSize', [ 8;],'ByteOrder', 'BigEndian','ValueType', 'UNSIGNED','Class', 'uint8','Signed', [ 0;],'Factor', [ 2;],'Offset', [ -500;],'Min', [ 0;],'Max', [ 0;],'Units', '','Comment', '','StartBit', [ 32;]),struct('Name', 'BP_OBU_Iregen_LC','Startbit', [ 0;],'SignalSize', [ 8;],'ByteOrder', 'BigEndian','ValueType', 'UNSIGNED','Class', 'uint8','Signed', [ 0;],'Factor', [ 2;],'Offset', [ 0;],'Min', [ 0;],'Max', [ 0;],'Units', '','Comment', '','StartBit', [ 40;]),struct('Name', 'BP_OBU_Ichg_EXP','Startbit', [ 0;],'SignalSize', [ 8;],'ByteOrder', 'BigEndian','ValueType', 'UNSIGNED','Class', 'uint8','Signed', [ 0;],'Factor', [ 0.5;],'Offset', [ 0;],'Min', [ 0;],'Max', [ 0;],'Units', '','Comment', '','StartBit', [ 48;]),struct('Name', 'BP_OBU_Vchg_EXP','Startbit', [ 0;],'SignalSize', [ 8;],'ByteOrder', 'BigEndian','ValueType', 'UNSIGNED','Class', 'uint8','Signed', [ 0;],'Factor', [ 0.5;],'Offset', [ 0;],'Min', [ 0;],'Max', [ 0;],'Units', '','Comment', '','StartBit', [ 56;])}}
      settings: SourceProductName=Raptor
  raptor_data_def1 : Raptor_lib/Data Storage/raptor_data_def  dataName='BP_OBU_Vmin_Limit'  initValue=0  dataType=double  storage=Volatile (RAM)  calVisible=on  calType=Measurement  calDispType=Number  calEnum={'False', 'True'}  calGain=1.0  calOffset=0  calMin=-inf  calMax=inf  calFormat='-1'  calUnit=''  calHelp=''  calAccess=1  calFunction=raptor_xcp_function(gcb)  calDispHeaders=off  calColHeaders={'Col1' 'Col2' 'Col3'}  calRowHeaders={'Row1' 'Row2' 'Row3'}
      settings: SourceProductName=Raptor
  raptor_data_def2 : Raptor_lib/Data Storage/raptor_data_def  dataName='BP_OBU_Vmax_Limit'  initValue=0  dataType=double  storage=Volatile (RAM)  calVisible=on  calType=Measurement  calDispType=Number  calEnum={'False', 'True'}  calGain=1.0  calOffset=0  calMin=-inf  calMax=inf  calFormat='-1'  calUnit=''  calHelp=''  calAccess=1  calFunction=raptor_xcp_function(gcb)  calDispHeaders=off  calColHeaders={'Col1' 'Col2' 'Col3'}  calRowHeaders={'Row1' 'Row2' 'Row3'}
      settings: SourceProductName=Raptor
  raptor_data_def4 : Raptor_lib/Data Storage/raptor_data_def  dataName='BP_OBU_Vchg_EXP'  initValue=0  dataType=double  storage=Volatile (RAM)  calVisible=on  calType=Measurement  calDispType=Number  calEnum={'False', 'True'}  calGain=1.0  calOffset=0  calMin=-inf  calMax=inf  calFormat='-1'  calUnit=''  calHelp=''  calAccess=1  calFunction=raptor_xcp_function(gcb)  calDispHeaders=off  calColHeaders={'Col1' 'Col2' 'Col3'}  calRowHeaders={'Row1' 'Row2' 'Row3'}
      settings: SourceProductName=Raptor
  raptor_data_read1 : Raptor_lib/Data Storage/raptor_data_read  dataName='Ichg_cc_exp'  dataShape=Scalar  idxSource=Input  idxRow=1  idxCol=1
      settings: SourceProductName=Raptor
  raptor_data_read2 : Raptor_lib/Data Storage/raptor_data_read  dataName='Iregen_con_exp'  dataShape=Scalar  idxSource=Input  idxRow=1  idxCol=1
      settings: SourceProductName=Raptor
  raptor_data_read3 : Raptor_lib/Data Storage/raptor_data_read  dataName='BP_OBU_Vchg_EXP'  dataShape=Scalar  idxSource=Input  idxRow=1  idxCol=1
      settings: SourceProductName=Raptor
  raptor_data_read4 : Raptor_lib/Data Storage/raptor_data_read  dataName='Idchg_con_exp'  dataShape=Scalar  idxSource=Input  idxRow=1  idxCol=1
      settings: SourceProductName=Raptor
  raptor_data_read5 : Raptor_lib/Data Storage/raptor_data_read  dataName='BP_OBU_Vmin_Limit'  dataShape=Scalar  idxSource=Input  idxRow=1  idxCol=1
      settings: SourceProductName=Raptor
  raptor_data_read6 : Raptor_lib/Data Storage/raptor_data_read  dataName='BP_OBU_Vmax_Limit'  dataShape=Scalar  idxSource=Input  idxRow=1  idxCol=1
      settings: SourceProductName=Raptor
  wires:
  raptor_data_read3/1 -> raptor_can_txmsg/1
  raptor_data_read1/1 -> raptor_can_txmsg/2
  raptor_data_read4/1 -> raptor_can_txmsg/4
  raptor_data_read5/1 -> raptor_can_txmsg/5
  raptor_data_read6/1 -> raptor_can_txmsg/6
  raptor_data_read2/1 -> raptor_can_txmsg/3

== system EPT/Foreground_TimeBase_5ms/CAN/CAN1_exec/BCU vs RMDA-BMS/BCU-OBU Output-EW Code ==
  Trigger : TriggerPort  VariantControl=Variant  PortDimensions=1
  raptor_can_txmsg : Raptor_lib/CAN/raptor_can_txmsg  canDefinition=struct('dbcFile', 'BCU_OBU_HMI.dbc','message', 'BCU_OBU_Output_EW_Code','comment', '','signals', {{'BP_OBU_Fault_G5','BP_OBU_Fault_G4','BP_OBU_Fault_G3','BP_OBU_Fault_G2','BP_OBU_Fault_G1','BP_OBU_Warning_G3','BP_OBU_Warning_G2','BP_OBU_Warning_G1'}},'enabled', [ 1 1 1 1 1 1 1 1;],'canBus', '''CAN1''','messageID', [ 1524;],'idMask', [ 536870911;],'payloadMask', [],'payloadValue', [],'period', [ 0;],'mailbox', '','queueSize', [ 1;],'label', [ 0;],'ver', [ 2;],'showID', [ 0;],'showRaw', [ 0;],'fill', [ 0;],'editID', [ 0;],'signalOrder', [ 2;])  canBus='CAN1'  queueSize=1  payloadMask=[]  payloadValue=[]  period=0  showID=0  label=0  idMask=hex2dec('1FFFFFFF')  fill=0  id=1524  showRaw=0  signalOrder=2  signalInfo={{struct('Name', 'BP_OBU_Warning_G3','Startbit', [ 0;],'SignalSize', [ 8;],'ByteOrder', 'BigEndian','ValueType', 'UNSIGNED','Class', 'uint8','Signed', [ 0;],'Factor', [ 1;],'Offset', [ 0;],'Min', [ 0;],'Max', [ 0;],'Units', '','Comment', '','StartBit', [ 16;]),struct('Name', 'BP_OBU_Warning_G2','Startbit', [ 0;],'SignalSize', [ 8;],'ByteOrder', 'BigEndian','ValueType', 'UNSIGNED','Class', 'uint8','Signed', [ 0;],'Factor', [ 1;],'Offset', [ 0;],'Min', [ 0;],'Max', [ 0;],'Units', '','Comment', '','StartBit', [ 8;]),struct('Name', 'BP_OBU_Warning_G1','Startbit', [ 0;],'SignalSize', [ 8;],'ByteOrder', 'BigEndian','ValueType', 'UNSIGNED','Class', 'uint8','Signed', [ 0;],'Factor', [ 1;],'Offset', [ 0;],'Min', [ 0;],'Max', [ 0;],'Units', '','Comment', '','StartBit', [ 0;]),struct('Name', 'BP_OBU_Fault_G5','Startbit', [ 0;],'SignalSize', [ 8;],'ByteOrder', 'BigEndian','ValueType', 'UNSIGNED','Class', 'uint8','Signed', [ 0;],'Factor', [ 1;],'Offset', [ 0;],'Min', [ 0;],'Max', [ 0;],'Units', '','Comment', '','StartBit', [ 56;]),struct('Name', 'BP_OBU_Fault_G4','Startbit', [ 0;],'SignalSize', [ 8;],'ByteOrder', 'BigEndian','ValueType', 'UNSIGNED','Class', 'uint8','Signed', [ 0;],'Factor', [ 1;],'Offset', [ 0;],'Min', [ 0;],'Max', [ 0;],'Units', '','Comment', '','StartBit', [ 48;]),struct('Name', 'BP_OBU_Fault_G3','Startbit', [ 0;],'SignalSize', [ 8;],'ByteOrder', 'BigEndian','ValueType', 'UNSIGNED','Class', 'uint8','Signed', [ 0;],'Factor', [ 1;],'Offset', [ 0;],'Min', [ 0;],'Max', [ 0;],'Units', '','Comment', '','StartBit', [ 40;]),struct('Name', 'BP_OBU_Fault_G2','Startbit', [ 0;],'SignalSize', [ 8;],'ByteOrder', 'BigEndian','ValueType', 'UNSIGNED','Class', 'uint8','Signed', [ 0;],'Factor', [ 1;],'Offset', [ 0;],'Min', [ 0;],'Max', [ 0;],'Units', '','Comment', '','StartBit', [ 32;]),struct('Name', 'BP_OBU_Fault_G1','Startbit', [ 0;],'SignalSize', [ 8;],'ByteOrder', 'BigEndian','ValueType', 'UNSIGNED','Class', 'uint8','Signed', [ 0;],'Factor', [ 1;],'Offset', [ 0;],'Min', [ 0;],'Max', [ 0;],'Units', '','Comment', '','StartBit', [ 24;])}}
      settings: SourceProductName=Raptor
  raptor_data_read : Raptor_lib/Data Storage/raptor_data_read  dataName='BP_OBU_Fault_G5'  dataShape=Scalar  idxSource=Input  idxRow=1  idxCol=1
      settings: SourceProductName=Raptor
  raptor_data_read1 : Raptor_lib/Data Storage/raptor_data_read  dataName='BP_OBU_Warning_G3'  dataShape=Scalar  idxSource=Input  idxRow=1  idxCol=1
      settings: SourceProductName=Raptor
  raptor_data_read2 : Raptor_lib/Data Storage/raptor_data_read  dataName='BP_OBU_Fault_G4'  dataShape=Scalar  idxSource=Input  idxRow=1  idxCol=1
      settings: SourceProductName=Raptor
  raptor_data_read3 : Raptor_lib/Data Storage/raptor_data_read  dataName='BP_OBU_Fault_G3'  dataShape=Scalar  idxSource=Input  idxRow=1  idxCol=1
      settings: SourceProductName=Raptor
  raptor_data_read4 : Raptor_lib/Data Storage/raptor_data_read  dataName='BP_OBU_Fault_G2'  dataShape=Scalar  idxSource=Input  idxRow=1  idxCol=1
      settings: SourceProductName=Raptor
  raptor_data_read5 : Raptor_lib/Data Storage/raptor_data_read  dataName='BP_OBU_Fault_G1'  dataShape=Scalar  idxSource=Input  idxRow=1  idxCol=1
      settings: SourceProductName=Raptor
  raptor_data_read6 : Raptor_lib/Data Storage/raptor_data_read  dataName='BP_OBU_Warning_G2'  dataShape=Scalar  idxSource=Input  idxRow=1  idxCol=1
      settings: SourceProductName=Raptor
  raptor_data_read7 : Raptor_lib/Data Storage/raptor_data_read  dataName='BP_OBU_Warning_G1'  dataShape=Scalar  idxSource=Input  idxRow=1  idxCol=1
      settings: SourceProductName=Raptor
  wires:
  raptor_data_read/1 -> raptor_can_txmsg/1
  raptor_data_read2/1 -> raptor_can_txmsg/2
  raptor_data_read3/1 -> raptor_can_txmsg/3
  raptor_data_read4/1 -> raptor_can_txmsg/4
  raptor_data_read5/1 -> raptor_can_txmsg/5
  raptor_data_read1/1 -> raptor_can_txmsg/6
  raptor_data_read6/1 -> raptor_can_txmsg/7
  raptor_data_read7/1 -> raptor_can_txmsg/8

== system EPT/Foreground_TimeBase_5ms/CAN/CAN1_exec/BCU vs RMDA-BMS/BCU-OBU Status-OP G1 ==
  Trigger : TriggerPort  VariantControl=Variant  PortDimensions=1
  raptor_can_txmsg : Raptor_lib/CAN/raptor_can_txmsg  canDefinition=struct('dbcFile', 'BCU_OBU_HMI.dbc','message', 'BCU_OBU_Status_OP_G1','comment', '','signals', {{'BP_OBU_Vbus','BP_OBU_Vbatt','BP_OBU_Current'}},'enabled', [ 1 1 1;],'canBus', '''CAN1''','messageID', [ 1525;],'idMask', [ 536870911;],'payloadMask', [],'payloadValue', [],'period', [ 0;],'mailbox', '','queueSize', [ 1;],'label', [ 0;],'ver', [ 2;],'showID', [ 0;],'showRaw', [ 0;],'fill', [ 0;],'editID', [ 0;],'signalOrder', [ 2;])  canBus='CAN1'  queueSize=1  payloadMask=[]  payloadValue=[]  period=0  showID=0  label=0  idMask=hex2dec('1FFFFFFF')  fill=0  id=1525  showRaw=0  signalOrder=2  signalInfo={{struct('Name', 'BP_OBU_Current','Startbit', [ 0;],'SignalSize', [ 16;],'ByteOrder', 'BigEndian','ValueType', 'UNSIGNED','Class', 'uint16','Signed', [ 0;],'Factor', [ 0.02;],'Offset', [ -500;],'Min', [ 0;],'Max', [ 0;],'Units', '','Comment', '','StartBit', [ 8;]),struct('Name', 'BP_OBU_Vbatt','Startbit', [ 0;],'SignalSize', [ 16;],'ByteOrder', 'BigEndian','ValueType', 'UNSIGNED','Class', 'uint16','Signed', [ 0;],'Factor', [ 0.01;],'Offset', [ 0;],'Min', [ 0;],'Max', [ 0;],'Units', '','Comment', '','StartBit', [ 24;]),struct('Name', 'BP_OBU_Vbus','Startbit', [ 0;],'SignalSize', [ 16;],'ByteOrder', 'BigEndian','ValueType', 'UNSIGNED','Class', 'uint16','Signed', [ 0;],'Factor', [ 0.01;],'Offset', [ 0;],'Min', [ 0;],'Max', [ 0;],'Units', '','Comment', '','StartBit', [ 40;])}}
      settings: SourceProductName=Raptor
  raptor_data_read1 : Raptor_lib/Data Storage/raptor_data_read  dataName='EPT_BPOBU_VOLT'  dataShape=Scalar  idxSource=Input  idxRow=1  idxCol=1
      settings: SourceProductName=Raptor
  raptor_data_read2 : Raptor_lib/Data Storage/raptor_data_read  dataName='EPT_HV_BUS_VOLT'  dataShape=Scalar  idxSource=Input  idxRow=1  idxCol=1
      settings: SourceProductName=Raptor
  raptor_data_read5 : Raptor_lib/Data Storage/raptor_data_read  dataName='EPT_BPOBU_CURR'  dataShape=Scalar  idxSource=Input  idxRow=1  idxCol=1
      settings: SourceProductName=Raptor
  wires:
  raptor_data_read2/1 -> raptor_can_txmsg/1
  raptor_data_read1/1 -> raptor_can_txmsg/2
  raptor_data_read5/1 -> raptor_can_txmsg/3
